simulink model "Simscape_crane_software_model_NPNC"  (R2016b)
settings: Solver=ode15s  StartTime=0.0  StopTime=120  RelTol=1e-3  EnableMultiTasking=on
values from neighbouring files (symbols this model uses):
  DC1x = 0.3    [RunModel.m]    (also in RunModelVerification.m)
  DC1y = 0.3    [RunModel.m]    (also in RunModelVerification.m)
  DC2x = 0.3    [RunModel.m]    (also in RunModelVerification.m)
  DC2y = 0.3    [RunModel.m]    (also in RunModelVerification.m)
  IC1x = 0.1    [RunModel.m]    (also in RunModelVerification.m)
  IC1y = 0.1    [RunModel.m]    (also in RunModelVerification.m)
  IC2x = 0.3    [RunModel.m]    (also in RunModelVerification.m)
  IC2y = 0.3    [RunModel.m]    (also in RunModelVerification.m)
  PC1x = 2.0    (= 2)    [RunModel.m]    (also in RunModelVerification.m)
  PC1y = 2.0    (= 2)    [RunModel.m]    (also in RunModelVerification.m)
  PC2x = 3.5    [RunModel.m]    (also in RunModelVerification.m)
  PC2y = 3.5    [RunModel.m]    (also in RunModelVerification.m)
  waypoints = [waypoints, find_nearest_obstacles(waypoints, Grid)]    [path_planning.m]    (also in path_to_waypoints.m = [])
undefined symbols (not defined in the file or in its folder): m, MR, TxBreak, TxCoulomb, TxVisc, TyBreak, TyCoulomb, TzBreak, TzCoulomb, X, xRange, xZero, Y, yRange, yZero, Z, zRange, zZero
undefined symbols (not defined in the file): M, TorqueMultX, TorqueMultY, TorqueMultZ, TxTrans, TyTrans, TyVisc, TzTrans, TzVisc
libraries: sm_lib x146, fl_lib x62, nesl_utility x24, simulink x14, elec_lib x9, sm_double_wishbone_suspension_lib x4, aerolibtransform2 x1
(part 15 of 15)

== system Simscape_crane_software_model_NPNC/Crane1/XY actuator/Y cart/CART/Motor ==
  MotorBlack : sm_lib/Body Elements/Solid  InertiaType=PointMass  Mass=0  MassUnits=kg  CenterOfMass=[0 0 0]  CenterOfMassUnits=m  MomentsOfInertia=[1 1 1]  MomentsOfInertiaUnits=kg*m^2  ProductsOfInertia=[0 0 0]  ProductsOfInertiaUnits=kg*m^2  DensityBased=off  Density=1000  DensityUnits=kg/(m^3)  DoExposeReferenceFrame=on  SerializedFrames=<Frames/>  GraphicType=FromGeometry  MarkerShape=Sphere  MarkerSize=10  MarkerSizeUnits=m  GraphicVisPropType=AdvancedVisualProperties  GraphicDiffuseColor=[0.1 0.1 0.0]  GraphicSpecularColor=[0.5 0.5 0.5 1.0]  GraphicAmbientColor=[0.15 0.2 0.3 1.0]  GraphicEmissiveColor=[0.0 0.0 0.0 1.0]  GraphicShininess=30  GraphicOpacity=1.0  GeometryShape=Cylinder  RectangleSize=[1 1]  RectangleSizeUnits=m  BrickDimensions=[0.06 0.12 0.12]  BrickDimensionUnits=m  CylinderRadius=1.7  CylinderRadiusUnits=cm  CylinderLength=6  CylinderLengthUnits=cm  SphereRadius=1  SphereRadiusUnits=m  EllipsoidRadii=[1 1 1]  EllipsoidRadiiUnits=m  ExtrusionCrossSection=[1 1; -1 1; -1 -1; 1 -1]  ExtrusionCrossSectionUnits=m  ExtrusionLength=1  ExtrusionLengthUnits=m  PolygonNumSides=3  PolygonOuterRadius=1  PolygonOuterRadiusUnits=m  ExtGeomFileType=STL  ExtGeomFileUnits=m  RevolutionCrossSection=[1 1; 1 -1; 2 -1; 2 1]  RevolutionCrossSectionUnits=m  RevolutionExtent=Full  RevolutionAngle=180  RevolutionAngleUnits=deg
  MotorGearbox : sm_lib/Body Elements/Solid  InertiaType=PointMass  Mass=0  MassUnits=kg  CenterOfMass=[0 0 0]  CenterOfMassUnits=m  MomentsOfInertia=[1 1 1]  MomentsOfInertiaUnits=kg*m^2  ProductsOfInertia=[0 0 0]  ProductsOfInertiaUnits=kg*m^2  DensityBased=off  Density=1000  DensityUnits=kg/(m^3)  DoExposeReferenceFrame=on  SerializedFrames=<Frames/>  GraphicType=FromGeometry  MarkerShape=Sphere  MarkerSize=10  MarkerSizeUnits=m  GraphicVisPropType=SimpleVisualProperties  GraphicDiffuseColor=[0.4 0.4 0.4]  GraphicSpecularColor=[0.5 0.5 0.5 1.0]  GraphicAmbientColor=[0.15 0.15 0.15 1.0]  GraphicEmissiveColor=[0.0 0.0 0.0 1.0]  GraphicShininess=75  GraphicOpacity=1.0  GeometryShape=Cylinder  RectangleSize=[1 1]  RectangleSizeUnits=m  BrickDimensions=[0.06 0.12 0.12]  BrickDimensionUnits=m  CylinderRadius=2.6  CylinderRadiusUnits=cm  CylinderLength=3  CylinderLengthUnits=cm  SphereRadius=1  SphereRadiusUnits=m  EllipsoidRadii=[1 1 1]  EllipsoidRadiiUnits=m  ExtrusionCrossSection=[1 1; -1 1; -1 -1; 1 -1]  ExtrusionCrossSectionUnits=m  ExtrusionLength=1  ExtrusionLengthUnits=m  PolygonNumSides=3  PolygonOuterRadius=1  PolygonOuterRadiusUnits=m  ExtGeomFileType=STL  ExtGeomFileUnits=m  RevolutionCrossSection=[1 1; 1 -1; 2 -1; 2 1]  RevolutionCrossSectionUnits=m  RevolutionExtent=Full  RevolutionAngle=180  RevolutionAngleUnits=deg
  Rigid Transform3 : sm_lib/Frames and Transforms/Rigid Transform  TranslationMethod=None  TranslationStandardOffset=0.04  TranslationLengthUnit=m  TranslationStandardAxis=-X  TranslationCartesianOffset="[-0.5 0  0]"  TranslationROffset=0  TranslationROffsetUnits=m  TranslationZOffset=0  TranslationZOffsetUnits=m  TranslationThetaOffset=0  TranslationThetaOffsetUnits=deg  RotationMethod=StandardAxis  RotationAngleUnits=deg  RotationStandardAxis=-X  RotationAngle=90  RotationArbitraryAxis=[0 0 1]  FollAlignAxisA=+X  BaseAlignAxisA=+Y  FollAlignAxisB=+Y  BaseAlignAxisB=+Z  RotationSequenceAxes=FollowerAxes  RotationSequence=XYX  RotationSequenceAngles=[0 0 0]  RotationSequenceAnglesUnits=deg  RotationMatrix=[1 0 0; 0 1 0; 0 0 1]
  Rigid Transform4 : sm_lib/Frames and Transforms/Rigid Transform  TranslationMethod=None  TranslationStandardOffset=0.04  TranslationLengthUnit=m  TranslationStandardAxis=-X  TranslationCartesianOffset="[-0.5 0  0]"  TranslationROffset=0  TranslationROffsetUnits=m  TranslationZOffset=0  TranslationZOffsetUnits=m  TranslationThetaOffset=0  TranslationThetaOffsetUnits=deg  RotationMethod=StandardAxis  RotationAngleUnits=deg  RotationStandardAxis=-X  RotationAngle=90  RotationArbitraryAxis=[0 0 1]  FollAlignAxisA=+X  BaseAlignAxisA=+Y  FollAlignAxisB=+Y  BaseAlignAxisB=+Z  RotationSequenceAxes=FollowerAxes  RotationSequence=XYX  RotationSequenceAngles=[0 0 0]  RotationSequenceAnglesUnits=deg  RotationMatrix=[1 0 0; 0 1 0; 0 0 1]
  Rigid Transform5 : sm_lib/Frames and Transforms/Rigid Transform  TranslationMethod=StandardAxis  TranslationStandardOffset=0.015  TranslationLengthUnit=m  TranslationStandardAxis=-Y  TranslationCartesianOffset="[-0.5 0  0]"  TranslationROffset=0  TranslationROffsetUnits=m  TranslationZOffset=0  TranslationZOffsetUnits=m  TranslationThetaOffset=0  TranslationThetaOffsetUnits=deg  RotationMethod=None  RotationAngleUnits=deg  RotationStandardAxis=-X  RotationAngle=90  RotationArbitraryAxis=[0 0 1]  FollAlignAxisA=+X  BaseAlignAxisA=+Y  FollAlignAxisB=+Y  BaseAlignAxisB=+Z  RotationSequenceAxes=FollowerAxes  RotationSequence=XYX  RotationSequenceAngles=[0 0 0]  RotationSequenceAnglesUnits=deg  RotationMatrix=[1 0 0; 0 1 0; 0 0 1]
  Rigid Transform6 : sm_lib/Frames and Transforms/Rigid Transform  TranslationMethod=StandardAxis  TranslationStandardOffset=0.03  TranslationLengthUnit=m  TranslationStandardAxis=+Y  TranslationCartesianOffset="[-0.5 0  0]"  TranslationROffset=0  TranslationROffsetUnits=m  TranslationZOffset=0  TranslationZOffsetUnits=m  TranslationThetaOffset=0  TranslationThetaOffsetUnits=deg  RotationMethod=None  RotationAngleUnits=deg  RotationStandardAxis=-X  RotationAngle=90  RotationArbitraryAxis=[0 0 1]  FollAlignAxisA=+X  BaseAlignAxisA=+Y  FollAlignAxisB=+Y  BaseAlignAxisB=+Z  RotationSequenceAxes=FollowerAxes  RotationSequence=XYX  RotationSequenceAngles=[0 0 0]  RotationSequenceAnglesUnits=deg  RotationMatrix=[1 0 0; 0 1 0; 0 0 1]
  Conn1 : PMIOPort  Port=1  Side=Left
  connections:
  Rigid Transform3/RConn1 -- MotorBlack/RConn1
  Rigid Transform4/RConn1 -- MotorGearbox/RConn1
  Rigid Transform6/LConn1 -- Conn1/RConn1 -- Rigid Transform5/LConn1
  Rigid Transform6/RConn1 -- Rigid Transform4/LConn1
  Rigid Transform5/RConn1 -- Rigid Transform3/LConn1

== system Simscape_crane_software_model_NPNC/Crane1/XY actuator/X rail/DC X/PWM & H-Bridge/PWM Scope ==
  Electrical Reference1 : fl_lib/Electrical/Electrical Elements/Electrical Reference
  PS-Simulink Converter 2 : nesl_utility/PS-Simulink Converter  PhysicalDomain=network_engine_domain  SubClassName=ps_output  LeftPortType=input  RightPortType=output  PseudoPeriodic=off  Frequencies=[]  Unit=V  AffineConversion=off
  PWM : Scope
  Voltage Sensor : fl_lib/Electrical/Electrical Sensors/Voltage Sensor
  u : PMIOPort  Port=1  Side=Left
  wires:
  PS-Simulink Converter 2/1 -> PWM/1
  connections:
  Voltage Sensor/RConn2 -- Electrical Reference1/LConn1
  Voltage Sensor/RConn1 -- PS-Simulink Converter 2/LConn1
  u/RConn1 -- Voltage Sensor/LConn1

== system Simscape_crane_software_model_NPNC/Crane1/XY actuator/X rail/DC X/PWM & H-Bridge/REV Scope ==
  Electrical Reference1 : fl_lib/Electrical/Electrical Elements/Electrical Reference
  PS-Simulink Converter 2 : nesl_utility/PS-Simulink Converter  PhysicalDomain=network_engine_domain  SubClassName=ps_output  LeftPortType=input  RightPortType=output  PseudoPeriodic=off  Frequencies=[]  Unit=V  AffineConversion=off
  REV : Scope
  Voltage Sensor : fl_lib/Electrical/Electrical Sensors/Voltage Sensor
  u : PMIOPort  Port=1  Side=Left
  wires:
  PS-Simulink Converter 2/1 -> REV/1
  connections:
  Voltage Sensor/RConn2 -- Electrical Reference1/LConn1
  Voltage Sensor/RConn1 -- PS-Simulink Converter 2/LConn1
  u/RConn1 -- Voltage Sensor/LConn1

== system Simscape_crane_software_model_NPNC/Crane1/XY actuator/X rail/DC X/PWM & H-Bridge/Vr Scope ==
  Electrical Reference1 : fl_lib/Electrical/Electrical Elements/Electrical Reference
  PS-Simulink Converter 2 : nesl_utility/PS-Simulink Converter  PhysicalDomain=network_engine_domain  SubClassName=ps_output  LeftPortType=input  RightPortType=output  PseudoPeriodic=off  Frequencies=[]  Unit=V  AffineConversion=off
  Voltage Sensor : fl_lib/Electrical/Electrical Sensors/Voltage Sensor
  Vr : Scope
  u : PMIOPort  Port=1  Side=Left
  wires:
  PS-Simulink Converter 2/1 -> Vr/1
  connections:
  u/RConn1 -- Voltage Sensor/LConn1
  Voltage Sensor/RConn1 -- PS-Simulink Converter 2/LConn1
  Voltage Sensor/RConn2 -- Electrical Reference1/LConn1

== system Simscape_crane_software_model_NPNC/Crane1/XY actuator/X rail/RAIL /Aesthetics/ClearPlastic ==
  Rail2 : sm_lib/Body Elements/Solid  InertiaType=PointMass  Mass=0  MassUnits=kg  CenterOfMass=[0 0 0]  CenterOfMassUnits=m  MomentsOfInertia=[1 1 1]  MomentsOfInertiaUnits=kg*m^2  ProductsOfInertia=[0 0 0]  ProductsOfInertiaUnits=kg*m^2  DensityBased=off  Density=1000  DensityUnits=kg/(m^3)  DoExposeReferenceFrame=on  SerializedFrames=<Frames/>  GraphicType=FromGeometry  MarkerShape=Sphere  MarkerSize=10  MarkerSizeUnits=m  GraphicVisPropType=SimpleVisualProperties  GraphicDiffuseColor=[0.8 0.8 0.8]  GraphicSpecularColor=[0.5 0.5 0.5 1.0]  GraphicAmbientColor=[0.15 0.15 0.15 1.0]  GraphicEmissiveColor=[0.0 0.0 0.0 1.0]  GraphicShininess=100  GraphicOpacity=0.4  GeometryShape=Brick  RectangleSize=[1 1]  RectangleSizeUnits=m  BrickDimensions=[0.05 0.09 0.015]  BrickDimensionUnits=m  CylinderRadius=0.02  CylinderRadiusUnits=m  CylinderLength=1  CylinderLengthUnits=m  SphereRadius=1  SphereRadiusUnits=m  EllipsoidRadii=[1 1 1]  EllipsoidRadiiUnits=m  ExtrusionCrossSection=[1 1; -1 1; -1 -1; 1 -1]  ExtrusionCrossSectionUnits=m  ExtrusionLength=1  ExtrusionLengthUnits=m  PolygonNumSides=3  PolygonOuterRadius=1  PolygonOuterRadiusUnits=m  ExtGeomFileType=STL  ExtGeomFileUnits=m  RevolutionCrossSection=[1 1; 1 -1; 2 -1; 2 1]  RevolutionCrossSectionUnits=m  RevolutionExtent=Full  RevolutionAngle=180  RevolutionAngleUnits=deg
  Rigid Transform11 : sm_lib/Frames and Transforms/Rigid Transform  TranslationMethod=None  TranslationStandardOffset=0.05  TranslationLengthUnit=m  TranslationStandardAxis=-Z  TranslationCartesianOffset="[-0.5 0  0]"  TranslationROffset=0  TranslationROffsetUnits=m  TranslationZOffset=0  TranslationZOffsetUnits=m  TranslationThetaOffset=0  TranslationThetaOffsetUnits=deg  RotationMethod=StandardAxis  RotationAngleUnits=deg  RotationStandardAxis=+Z  RotationAngle=90  RotationArbitraryAxis=[0 0 1]  FollAlignAxisA=+X  BaseAlignAxisA=+Y  FollAlignAxisB=+Y  BaseAlignAxisB=+Z  RotationSequenceAxes=FollowerAxes  RotationSequence=XYX  RotationSequenceAngles=[0 0 0]  RotationSequenceAnglesUnits=deg  RotationMatrix=[1 0 0; 0 1 0; 0 0 1]
  Rigid Transform12 : sm_lib/Frames and Transforms/Rigid Transform  TranslationMethod=StandardAxis  TranslationStandardOffset=0.03  TranslationLengthUnit=m  TranslationStandardAxis=-X  TranslationCartesianOffset="[-0.5 0  0]"  TranslationROffset=0  TranslationROffsetUnits=m  TranslationZOffset=0  TranslationZOffsetUnits=m  TranslationThetaOffset=0  TranslationThetaOffsetUnits=deg  RotationMethod=None  RotationAngleUnits=deg  RotationStandardAxis=+Y  RotationAngle=90  RotationArbitraryAxis=[0 0 1]  FollAlignAxisA=+X  BaseAlignAxisA=+Y  FollAlignAxisB=+Y  BaseAlignAxisB=+Z  RotationSequenceAxes=FollowerAxes  RotationSequence=XYX  RotationSequenceAngles=[0 0 0]  RotationSequenceAnglesUnits=deg  RotationMatrix=[1 0 0; 0 1 0; 0 0 1]
  Rigid Transform8 : sm_lib/Frames and Transforms/Rigid Transform  TranslationMethod=None  TranslationStandardOffset=0.05  TranslationLengthUnit=m  TranslationStandardAxis=-Z  TranslationCartesianOffset="[-0.5 0  0]"  TranslationROffset=0  TranslationROffsetUnits=m  TranslationZOffset=0  TranslationZOffsetUnits=m  TranslationThetaOffset=0  TranslationThetaOffsetUnits=deg  RotationMethod=StandardAxis  RotationAngleUnits=deg  RotationStandardAxis=+X  RotationAngle=90  RotationArbitraryAxis=[0 0 1]  FollAlignAxisA=+X  BaseAlignAxisA=+Y  FollAlignAxisB=+Y  BaseAlignAxisB=+Z  RotationSequenceAxes=FollowerAxes  RotationSequence=XYX  RotationSequenceAngles=[0 0 0]  RotationSequenceAnglesUnits=deg  RotationMatrix=[1 0 0; 0 1 0; 0 0 1]
  Conn1 : PMIOPort  Port=1  Side=Right
  connections:
  Rigid Transform12/LConn1 -- Conn1/RConn1
  Rigid Transform8/LConn1 -- Rigid Transform11/RConn1
  Rigid Transform11/LConn1 -- Rigid Transform12/RConn1
  Rigid Transform8/RConn1 -- Rail2/RConn1

== system Simscape_crane_software_model_NPNC/Crane1/XY actuator/X rail/RAIL /Aesthetics/ClearPlastic1 ==
  Rail2 : sm_lib/Body Elements/Solid  InertiaType=PointMass  Mass=0  MassUnits=kg  CenterOfMass=[0 0 0]  CenterOfMassUnits=m  MomentsOfInertia=[1 1 1]  MomentsOfInertiaUnits=kg*m^2  ProductsOfInertia=[0 0 0]  ProductsOfInertiaUnits=kg*m^2  DensityBased=off  Density=1000  DensityUnits=kg/(m^3)  DoExposeReferenceFrame=on  SerializedFrames=<Frames/>  GraphicType=FromGeometry  MarkerShape=Sphere  MarkerSize=10  MarkerSizeUnits=m  GraphicVisPropType=SimpleVisualProperties  GraphicDiffuseColor=[0.8 0.8 0.8]  GraphicSpecularColor=[0.5 0.5 0.5 1.0]  GraphicAmbientColor=[0.15 0.15 0.15 1.0]  GraphicEmissiveColor=[0.0 0.0 0.0 1.0]  GraphicShininess=100  GraphicOpacity=0.4  GeometryShape=Brick  RectangleSize=[1 1]  RectangleSizeUnits=m  BrickDimensions=[0.05 0.09 0.015]  BrickDimensionUnits=m  CylinderRadius=0.02  CylinderRadiusUnits=m  CylinderLength=1  CylinderLengthUnits=m  SphereRadius=1  SphereRadiusUnits=m  EllipsoidRadii=[1 1 1]  EllipsoidRadiiUnits=m  ExtrusionCrossSection=[1 1; -1 1; -1 -1; 1 -1]  ExtrusionCrossSectionUnits=m  ExtrusionLength=1  ExtrusionLengthUnits=m  PolygonNumSides=3  PolygonOuterRadius=1  PolygonOuterRadiusUnits=m  ExtGeomFileType=STL  ExtGeomFileUnits=m  RevolutionCrossSection=[1 1; 1 -1; 2 -1; 2 1]  RevolutionCrossSectionUnits=m  RevolutionExtent=Full  RevolutionAngle=180  RevolutionAngleUnits=deg
  Rigid Transform11 : sm_lib/Frames and Transforms/Rigid Transform  TranslationMethod=None  TranslationStandardOffset=0.05  TranslationLengthUnit=m  TranslationStandardAxis=-Z  TranslationCartesianOffset="[-0.5 0  0]"  TranslationROffset=0  TranslationROffsetUnits=m  TranslationZOffset=0  TranslationZOffsetUnits=m  TranslationThetaOffset=0  TranslationThetaOffsetUnits=deg  RotationMethod=StandardAxis  RotationAngleUnits=deg  RotationStandardAxis=+Z  RotationAngle=90  RotationArbitraryAxis=[0 0 1]  FollAlignAxisA=+X  BaseAlignAxisA=+Y  FollAlignAxisB=+Y  BaseAlignAxisB=+Z  RotationSequenceAxes=FollowerAxes  RotationSequence=XYX  RotationSequenceAngles=[0 0 0]  RotationSequenceAnglesUnits=deg  RotationMatrix=[1 0 0; 0 1 0; 0 0 1]
  Rigid Transform12 : sm_lib/Frames and Transforms/Rigid Transform  TranslationMethod=StandardAxis  TranslationStandardOffset=0.03  TranslationLengthUnit=m  TranslationStandardAxis=-X  TranslationCartesianOffset="[-0.5 0  0]"  TranslationROffset=0  TranslationROffsetUnits=m  TranslationZOffset=0  TranslationZOffsetUnits=m  TranslationThetaOffset=0  TranslationThetaOffsetUnits=deg  RotationMethod=None  RotationAngleUnits=deg  RotationStandardAxis=+Y  RotationAngle=90  RotationArbitraryAxis=[0 0 1]  FollAlignAxisA=+X  BaseAlignAxisA=+Y  FollAlignAxisB=+Y  BaseAlignAxisB=+Z  RotationSequenceAxes=FollowerAxes  RotationSequence=XYX  RotationSequenceAngles=[0 0 0]  RotationSequenceAnglesUnits=deg  RotationMatrix=[1 0 0; 0 1 0; 0 0 1]
  Rigid Transform8 : sm_lib/Frames and Transforms/Rigid Transform  TranslationMethod=None  TranslationStandardOffset=0.05  TranslationLengthUnit=m  TranslationStandardAxis=-Z  TranslationCartesianOffset="[-0.5 0  0]"  TranslationROffset=0  TranslationROffsetUnits=m  TranslationZOffset=0  TranslationZOffsetUnits=m  TranslationThetaOffset=0  TranslationThetaOffsetUnits=deg  RotationMethod=StandardAxis  RotationAngleUnits=deg  RotationStandardAxis=+X  RotationAngle=90  RotationArbitraryAxis=[0 0 1]  FollAlignAxisA=+X  BaseAlignAxisA=+Y  FollAlignAxisB=+Y  BaseAlignAxisB=+Z  RotationSequenceAxes=FollowerAxes  RotationSequence=XYX  RotationSequenceAngles=[0 0 0]  RotationSequenceAnglesUnits=deg  RotationMatrix=[1 0 0; 0 1 0; 0 0 1]
  Conn1 : PMIOPort  Port=1  Side=Right
  connections:
  Rigid Transform8/RConn1 -- Rail2/RConn1
  Rigid Transform11/LConn1 -- Rigid Transform12/RConn1
  Rigid Transform8/LConn1 -- Rigid Transform11/RConn1
  Rigid Transform12/LConn1 -- Conn1/RConn1

== system Simscape_crane_software_model_NPNC/Crane1/XY actuator/X rail/RAIL /Aesthetics/Motor ==
  MotorGearbox : sm_lib/Body Elements/Solid  InertiaType=PointMass  Mass=0  MassUnits=kg  CenterOfMass=[0 0 0]  CenterOfMassUnits=m  MomentsOfInertia=[1 1 1]  MomentsOfInertiaUnits=kg*m^2  ProductsOfInertia=[0 0 0]  ProductsOfInertiaUnits=kg*m^2  DensityBased=off  Density=1000  DensityUnits=kg/(m^3)  DoExposeReferenceFrame=on  SerializedFrames=<Frames/>  GraphicType=FromGeometry  MarkerShape=Sphere  MarkerSize=10  MarkerSizeUnits=m  GraphicVisPropType=SimpleVisualProperties  GraphicDiffuseColor=[0.4 0.4 0.4]  GraphicSpecularColor=[0.5 0.5 0.5 1.0]  GraphicAmbientColor=[0.15 0.15 0.15 1.0]  GraphicEmissiveColor=[0.0 0.0 0.0 1.0]  GraphicShininess=75  GraphicOpacity=1.0  GeometryShape=Cylinder  RectangleSize=[1 1]  RectangleSizeUnits=m  BrickDimensions=[0.06 0.12 0.12]  BrickDimensionUnits=m  CylinderRadius=2.6  CylinderRadiusUnits=cm  CylinderLength=3  CylinderLengthUnits=cm  SphereRadius=1  SphereRadiusUnits=m  EllipsoidRadii=[1 1 1]  EllipsoidRadiiUnits=m  ExtrusionCrossSection=[1 1; -1 1; -1 -1; 1 -1]  ExtrusionCrossSectionUnits=m  ExtrusionLength=1  ExtrusionLengthUnits=m  PolygonNumSides=3  PolygonOuterRadius=1  PolygonOuterRadiusUnits=m  ExtGeomFileType=STL  ExtGeomFileUnits=m  RevolutionCrossSection=[1 1; 1 -1; 2 -1; 2 1]  RevolutionCrossSectionUnits=m  RevolutionExtent=Full  RevolutionAngle=180  RevolutionAngleUnits=deg
  Rigid Transform3 : sm_lib/Frames and Transforms/Rigid Transform  TranslationMethod=None  TranslationStandardOffset=0.04  TranslationLengthUnit=m  TranslationStandardAxis=-X  TranslationCartesianOffset="[-0.5 0  0]"  TranslationROffset=0  TranslationROffsetUnits=m  TranslationZOffset=0  TranslationZOffsetUnits=m  TranslationThetaOffset=0  TranslationThetaOffsetUnits=deg  RotationMethod=StandardAxis  RotationAngleUnits=deg  RotationStandardAxis=-X  RotationAngle=90  RotationArbitraryAxis=[0 0 1]  FollAlignAxisA=+X  BaseAlignAxisA=+Y  FollAlignAxisB=+Y  BaseAlignAxisB=+Z  RotationSequenceAxes=FollowerAxes  RotationSequence=XYX  RotationSequenceAngles=[0 0 0]  RotationSequenceAnglesUnits=deg  RotationMatrix=[1 0 0; 0 1 0; 0 0 1]
  Rigid Transform4 : sm_lib/Frames and Transforms/Rigid Transform  TranslationMethod=None  TranslationStandardOffset=0.04  TranslationLengthUnit=m  TranslationStandardAxis=-X  TranslationCartesianOffset="[-0.5 0  0]"  TranslationROffset=0  TranslationROffsetUnits=m  TranslationZOffset=0  TranslationZOffsetUnits=m  TranslationThetaOffset=0  TranslationThetaOffsetUnits=deg  RotationMethod=StandardAxis  RotationAngleUnits=deg  RotationStandardAxis=-X  RotationAngle=90  RotationArbitraryAxis=[0 0 1]  FollAlignAxisA=+X  BaseAlignAxisA=+Y  FollAlignAxisB=+Y  BaseAlignAxisB=+Z  RotationSequenceAxes=FollowerAxes  RotationSequence=XYX  RotationSequenceAngles=[0 0 0]  RotationSequenceAnglesUnits=deg  RotationMatrix=[1 0 0; 0 1 0; 0 0 1]
  Rigid Transform5 : sm_lib/Frames and Transforms/Rigid Transform  TranslationMethod=StandardAxis  TranslationStandardOffset=0.015  TranslationLengthUnit=m  TranslationStandardAxis=-Y  TranslationCartesianOffset="[-0.5 0  0]"  TranslationROffset=0  TranslationROffsetUnits=m  TranslationZOffset=0  TranslationZOffsetUnits=m  TranslationThetaOffset=0  TranslationThetaOffsetUnits=deg  RotationMethod=None  RotationAngleUnits=deg  RotationStandardAxis=-X  RotationAngle=90  RotationArbitraryAxis=[0 0 1]  FollAlignAxisA=+X  BaseAlignAxisA=+Y  FollAlignAxisB=+Y  BaseAlignAxisB=+Z  RotationSequenceAxes=FollowerAxes  RotationSequence=XYX  RotationSequenceAngles=[0 0 0]  RotationSequenceAnglesUnits=deg  RotationMatrix=[1 0 0; 0 1 0; 0 0 1]
  Rigid Transform6 : sm_lib/Frames and Transforms/Rigid Transform  TranslationMethod=StandardAxis  TranslationStandardOffset=0.03  TranslationLengthUnit=m  TranslationStandardAxis=+Y  TranslationCartesianOffset="[-0.5 0  0]"  TranslationROffset=0  TranslationROffsetUnits=m  TranslationZOffset=0  TranslationZOffsetUnits=m  TranslationThetaOffset=0  TranslationThetaOffsetUnits=deg  RotationMethod=None  RotationAngleUnits=deg  RotationStandardAxis=-X  RotationAngle=90  RotationArbitraryAxis=[0 0 1]  FollAlignAxisA=+X  BaseAlignAxisA=+Y  FollAlignAxisB=+Y  BaseAlignAxisB=+Z  RotationSequenceAxes=FollowerAxes  RotationSequence=XYX  RotationSequenceAngles=[0 0 0]  RotationSequenceAnglesUnits=deg  RotationMatrix=[1 0 0; 0 1 0; 0 0 1]
  motorBlack : sm_lib/Body Elements/Solid  InertiaType=PointMass  Mass=0  MassUnits=kg  CenterOfMass=[0 0 0]  CenterOfMassUnits=m  MomentsOfInertia=[1 1 1]  MomentsOfInertiaUnits=kg*m^2  ProductsOfInertia=[0 0 0]  ProductsOfInertiaUnits=kg*m^2  DensityBased=off  Density=1000  DensityUnits=kg/(m^3)  DoExposeReferenceFrame=on  SerializedFrames=<Frames/>  GraphicType=FromGeometry  MarkerShape=Sphere  MarkerSize=10  MarkerSizeUnits=m  GraphicVisPropType=AdvancedVisualProperties  GraphicDiffuseColor=[0.1 0.1 0.0]  GraphicSpecularColor=[0.5 0.5 0.5 1.0]  GraphicAmbientColor=[0.15 0.2 0.3 1.0]  GraphicEmissiveColor=[0.0 0.0 0.0 1.0]  GraphicShininess=30  GraphicOpacity=1.0  GeometryShape=Cylinder  RectangleSize=[1 1]  RectangleSizeUnits=m  BrickDimensions=[0.06 0.12 0.12]  BrickDimensionUnits=m  CylinderRadius=1.7  CylinderRadiusUnits=cm  CylinderLength=6  CylinderLengthUnits=cm  SphereRadius=1  SphereRadiusUnits=m  EllipsoidRadii=[1 1 1]  EllipsoidRadiiUnits=m  ExtrusionCrossSection=[1 1; -1 1; -1 -1; 1 -1]  ExtrusionCrossSectionUnits=m  ExtrusionLength=1  ExtrusionLengthUnits=m  PolygonNumSides=3  PolygonOuterRadius=1  PolygonOuterRadiusUnits=m  ExtGeomFileType=STL  ExtGeomFileUnits=m  RevolutionCrossSection=[1 1; 1 -1; 2 -1; 2 1]  RevolutionCrossSectionUnits=m  RevolutionExtent=Full  RevolutionAngle=180  RevolutionAngleUnits=deg
  Conn1 : PMIOPort  Port=1  Side=Left
  connections:
  Rigid Transform3/RConn1 -- motorBlack/RConn1
  Rigid Transform4/RConn1 -- MotorGearbox/RConn1
  Rigid Transform5/LConn1 -- Rigid Transform6/LConn1 -- Conn1/RConn1
  Rigid Transform6/RConn1 -- Rigid Transform4/LConn1
  Rigid Transform5/RConn1 -- Rigid Transform3/LConn1

== matlab function Simscape_crane_software_model_NPNC/Select most convenient path1 ==
  data: x output; y output; x_pos input; y_pos input; Waypoints input; Class output
function [x,y, Class] = Path_Selector(x_pos, y_pos, Waypoints)
persistent WP_Index

if isempty(WP_Index)
    WP_Index = 1;
end

Class = 1;

%% Random default values - dont touch
x = 0.252;
y = 0.365;
if WP_Index <= (length(Waypoints))
    x = Waypoints(WP_Index,1)/100;
    y = Waypoints(WP_Index,2)/100;
    
    %% Establish boundary conditions and controller class
    x_max = x+0.02;
    x_min = x-0.02;
    y_max = y+0.02;
    y_min = y-0.02;
    
    Class = 4;
    if distance(x,y, Waypoints(WP_Index,3), Waypoints(WP_Index,4)) < 0.1
        Class = 3;
    end
    
    if Waypoints(WP_Index,5) == 1
        x_max = x+0.01;
        x_min = x-0.01;
        y_max = y+0.01;
        y_min = y-0.01;
    
        Class = 2;
        if abs(distance(x,y,x_pos,y_pos)) < 0.1
            Class = 1;
        end
    end
    
    
    %% Crane arrived to point
    if (((x_pos <= x_max) && (x_pos >= x_min)) && ((y_pos <= y_max) && (y_pos >= y_min)))
        WP_Index = WP_Index + 1; 
        if WP_Index > (length(Waypoints))
            WP_Index = WP_Index - 1;
        end
    end
end

== matlab function Simscape_crane_software_model_NPNC/Controller1/Enforce Soft Limits and Overflow ==
  data: x input; u_x output; y input; u_x_in input; u_y_in input; x_Range input; y_Range input; u_y output
function [u_x, u_y] = fcn(x, y, u_x_in, u_y_in, x_Range, y_Range)

buff_up = 0.08;
buff_low = 0.08;
u_x = u_x_in;
u_y = u_y_in;

% Deal with overflow - may not be the most appropriate place
if(x > 10 || x < -10)
   x = 0;
end
if (y > 10 || y < -10)
   y = 0;
end

% Put in place soft boundaries on the borders
if (x > (x_Range(2)-buff_up))
    u_x = min(u_x_in,0);
end

if (x < (x_Range(1)+buff_low))
    u_x = max(u_x_in,0);
end


if (y > (y_Range(2)-buff_up))
    u_y = min(u_y_in,0);
end

if (y < (y_Range(1)+buff_low))
    u_y = max(u_y_in,0);
end


end

== matlab function Simscape_crane_software_model_NPNC/Controller1/PID Controler/GainDesch ==
  data: C1 input; Out output; C2 input; C3 input; C4 input; Class input
function Out = Demux(C1,C2, C3, C4, Class)

Out = C1;

switch Class
    case 1
        Out = C1;
    case 2
        Out = C2;
    case 3
        Out = C3;
    case 4
        Out = C4;
end

== matlab function Simscape_crane_software_model_NPNC/Controller1/PID Controler/GainDesch1 ==
  data: C1 input; Out output; C2 input; C3 input; C4 input; Class input
function Out = Demux(C1,C2, C3, C4, Class)

Out = C1;

switch Class
    case 1
        Out = C1;
    case 2
        Out = C2;
    case 3
        Out = C3;
    case 4
        Out = C4;
end

== matlab function Simscape_crane_software_model_NPNC/Controller1/PID Controler/GainSch ==
  data: Input input; C1 output; Class input; C2 output; C3 output; C4 output
function [C1,C2,C3,C4] = ContrMux(Input, Class)

C1 = 0;
C2 = 0;
C3 = 0;
C4 = 0;

switch Class
    case 1
        C1 = Input;
    case 2
        C2 = Input;
    case 3
        C3 = Input;
    case 4
        C4 = Input;
end

== matlab function Simscape_crane_software_model_NPNC/Controller1/PID Controler/GainSch1 ==
  data: Input input; C1 output; Class input; C2 output; C3 output; C4 output
function [C1,C2,C3,C4] = ContrMux(Input, Class)

C1 = 0;
C2 = 0;
C3 = 0;
C4 = 0;

switch Class
    case 1
        C1 = Input;
    case 2
        C2 = Input;
    case 3
        C3 = Input;
    case 4
        C4 = Input;
end

== matlab function Simscape_crane_software_model_NPNC/Convert Coordinates1 ==
  data: x output; y output; x_out input; y_out input; alpha_out input; beta_out input
function [x,y] = Sensors2World(x_out,y_out,alpha_out, beta_out)

%% Assumptions
R = 0.3;

%% Obtain Measurements from sensors
now_x = x_out;
now_y = y_out;
now_alpha = alpha_out + pi/2;
now_beta = beta_out;

sin_a = sin(now_alpha);
sin_b = sin(now_beta);
cos_a = cos(now_alpha);

x = now_x + R * sin_a * sin_b;
y = now_y + R * cos_a;
